simulink model "cec_ut"  (Simulink 8.1)
settings: Solver=FixedStepDiscrete  StartTime=0.0  StopTime=Inf  FixedStep=0.005  RelTol=1e-3
PostLoadFcn:
  | , if any(exist('dsrtsu_mdlpostloadfcn', 'file') == [2, 3, 6]), try dsrtsu_mdlpostloadfcn('Execute', bdroot); catch fprintf('Error in PostLoadFcn (dsrtsu_mdlpostloadfcn) for model "%s":\n %s\n', bdroot, lasterr); end, end,
libraries: siltestlib x10, cec x1
settings Model: DSRTSU_INTERNAL_RTI_VER=450  DSRTSU_INTERNAL_RTI_TYPE=rti1401  RTICANMMDATA=struct('GeneralSetupData',struct('modelroot','D:\ELN150201_TAIWAN\trunk\AdasDragon\software\sw_development\arch\app\jud','generalsettings',struct('filesettings',struct('destfolder',struct('Name','RTICANMM_FILES','Check',1),'buildfolder',struct('Name','.','Check',1),'AbsDestfolder',struct('Name','D:\ELN150201_TAIWAN\trunk\AdasDragon\software\sw_development\arch\app\jud\RTICANMM_FILES'),'AbsBuildfolder',struct('Name','D:\ELN150201_TAIWAN\trunk\AdasDragon\software\sw_development\arch\app\jud'))),'options',struct('addpaths',1,'rmpaths',1,'addtrcexclusion',logical(1),'cannavigator',struct('checkmonitoring',0),'show_usrtrc',0,'use_usrtrc',0),'advanced',struct('options',[1 1 1 1 1 1 1 1 1 1 1 1 1 1 1 1 1 1 1 1 1 1 1 1 1 1 1 1 1 1 1 1 1 1 1 1 1 1 1 1 1 1 1 1 1 1 1 1 1 1 1 1 1 1 1 1 1 1 1 1 1 1 1 1 1 1 1 1 1 1 1 1 1 1 1 1 1 1 1 1 1 1 1 1 1 1 1 1 1 1 1 1 1 1 1 1 1 1 1 1]),'MPSetup',{{}},'modelname','cec_ut','block','cec_ut'))  DSRTSU_INTERNAL_RTIFPGA=40  Creator=AT015411  LastModifiedBy=AT015555  BufferReuse=off
settings DataIOCC: SignalLoggingSaveFormat=Dataset
settings OptimizationCC: BlockReduction=off  OptimizeBlockIOStorage=off  BufferReuse=off  ExpressionFolding=off  ExpressionDepthLimit=128  LocalBlockOutputs=off
settings DebuggingCC: FcnCallInpInsideContextMsg=EnableAllAsError
settings HardwareCC: ProdIntDivRoundTo=Zero  ProdEndianess=BigEndian  ProdHWDeviceType=Generic->Custom  TargetIntDivRoundTo=Zero  TargetEndianess=BigEndian  TargetHWDeviceType=Generic->Custom
settings RTWCC: SystemTargetFile=rti1005.tlc  MakeCommand=make_rti  TemplateMakefile=rti1005.tmf  Description=dSPACE DS1005 Hardware Platform  ProcessScript=rti1005_make_rtw_hook
settings STFCustomTargetCC: CodeReplacementLibrary=ANSI_C  ParMdlRefBuildCompliant=on  GeneratePreprocessorConditionals=Disable all  MatFileLogging=on  SystemTargetFile=rti1005.tlc
settings GRTTargetCC: CompOptLevelCompliant=off  ConcurrentExecutionCompliant=off  ExtModeMexFile=noextcomm
settings CustomProperty: DataType=RTWOptions_EnumType_C__Program Files (x86)_dSPACE RCPHIL 2014-B_MATLAB_RTI_RTI1401_TLC_rti1005_1InitialSimState  Value=RUN
settings EnumStrPairs: String=RUN

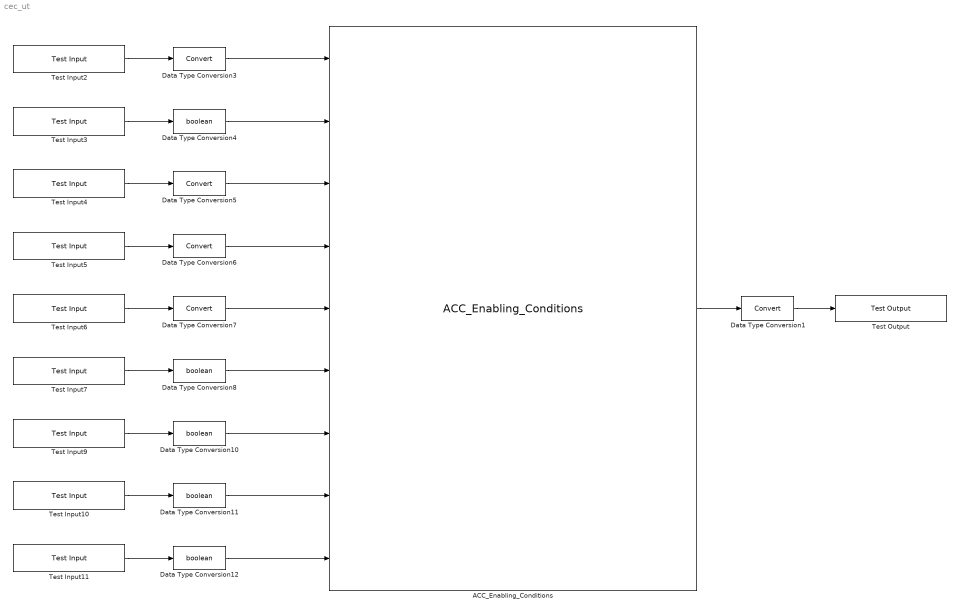
== system cec_ut ==
  ACC_Enabling_Conditions : cec/ACC_Enabling_Conditions
  Data Type Conversion{1,3,5..7} (5 alike) : DataTypeConversion
  Data Type Conversion{4,8,10..12} (5 alike) : DataTypeConversion  OutDataTypeStr=boolean
  Test Input10 : siltestlib/Test Input  varname=VDHP_DisableACC_flg  sampletime=0.005
  Test Input11 : siltestlib/Test Input  varname=VDINR_DriverBrakPedalOn_flg  sampletime=0.005
  Test Input2 : siltestlib/Test Input  varname=VDINR_KeySwitchStatus_enum  sampletime=0.005
  Test Input3 : siltestlib/Test Input  varname=VDINR_HMICANValid_flg  sampletime=0.005
  Test Input4 : siltestlib/Test Input  varname=VPER_CameraStatus_enum  sampletime=0.005
  Test Input5 : siltestlib/Test Input  varname=VPER_RadarStatus_enum  sampletime=0.005
  Test Input6 : siltestlib/Test Input  varname=VPER_FusionStatus_enum  sampletime=0.005
  Test Input7 : siltestlib/Test Input  varname=VIFO_VehicleStatusOk_flg  sampletime=0.005
  Test Input9 : siltestlib/Test Input  varname=VDHP_DisableADASFun_flg  sampletime=0.005
  Test Output : siltestlib/Test Output  varname=VJUD_ACCEnableReq_flg  sampletime=-1
  wires:
  Data Type Conversion1/1 -> Test Output/1
  Test Input2/1 -> Data Type Conversion3/1
  Test Input3/1 -> Data Type Conversion4/1
  Data Type Conversion3/1 -> ACC_Enabling_Conditions/1
  Data Type Conversion4/1 -> ACC_Enabling_Conditions/2
  Test Input4/1 -> Data Type Conversion5/1
  Test Input5/1 -> Data Type Conversion6/1
  Test Input6/1 -> Data Type Conversion7/1
  Test Input7/1 -> Data Type Conversion8/1
  Data Type Conversion5/1 -> ACC_Enabling_Conditions/3
  Data Type Conversion6/1 -> ACC_Enabling_Conditions/4
  Data Type Conversion7/1 -> ACC_Enabling_Conditions/5
  Data Type Conversion8/1 -> ACC_Enabling_Conditions/6
  Test Input9/1 -> Data Type Conversion10/1
  Test Input10/1 -> Data Type Conversion11/1
  Test Input11/1 -> Data Type Conversion12/1
  Data Type Conversion10/1 -> ACC_Enabling_Conditions/7
  Data Type Conversion11/1 -> ACC_Enabling_Conditions/8
  Data Type Conversion12/1 -> ACC_Enabling_Conditions/9
  ACC_Enabling_Conditions/1 -> Data Type Conversion1/1
